simulink model "NL1model"  (R2024a)
settings: Solver=FixedStepAuto  StartTime=0.0  StopTime=100  FixedStep=0.001  RelTol=1e-3  AbsTol=1e-3
libraries: fl_lib x17, nesl_utility x11, simulink x3, sdl_lib x1
settings Model: Creator=sa21280  LastModifiedBy=sa21280
settings SolverCC: AutoScaleAbsTol=off  AlgebraicLoopSolver=TrustRegion  MaxZcPerStep=1
settings DebuggingCC: UnconnectedInputMsg=warning  UnconnectedOutputMsg=warning  UnconnectedLineMsg=warning  SymbolicDimsDataTypeCodeGenerationDiagnostic=none
settings ModelReferenceCC: EnableRefExpFcnMdlSchedulingChecks=on
settings SFSimCC: CustomCodeUndefinedFunction=UseInterfaceOnly
settings RTWCC: GPUComputeCapability=3.5  DLArmComputeVersion=19.05
settings SimscapeCC: SimscapeLogType=all  SimscapeLogSimulationStatistics=on  SimscapeLogDataHistory=10000

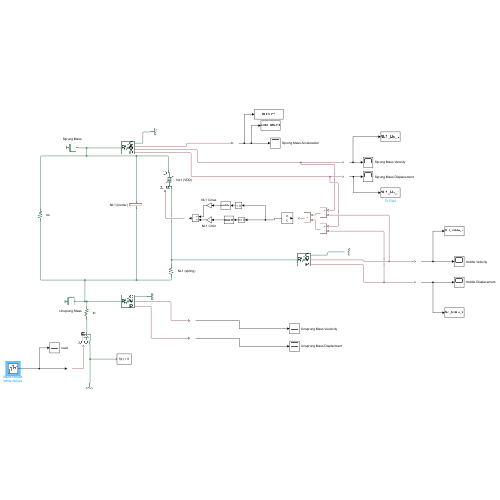
[thumbnail: Simulink's stored preview of the top-level diagram]
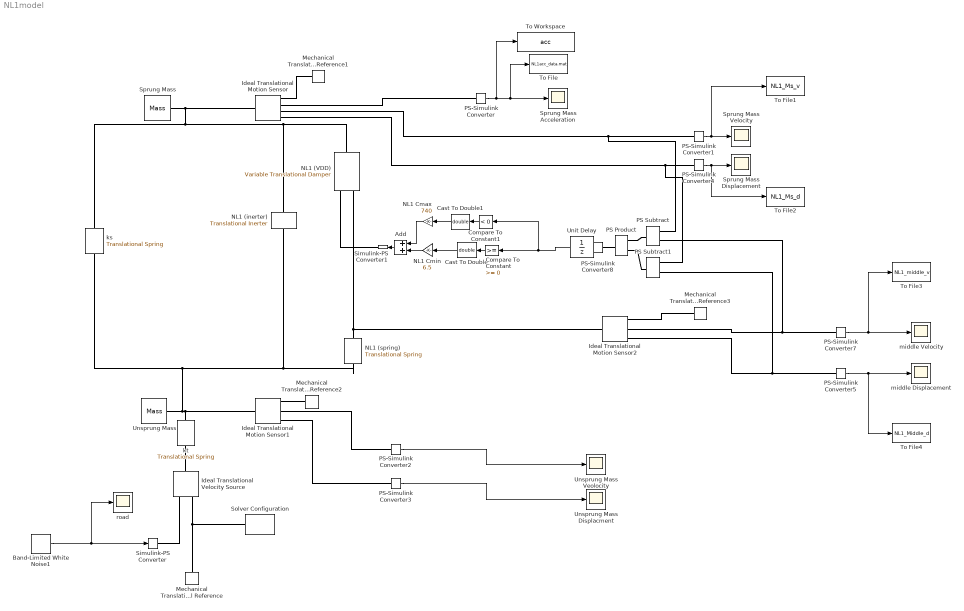
== system NL1model ==
  Add : Sum
  Band-Limited White Noise1 : simulink/Sources/Band-Limited White Noise  Cov=(2*pi*(25*5e-7).^0.5).^2  Ts=0.001  seed=[23341]
  Cast To Double : DataTypeConversion  OutDataTypeStr=double  SaturateOnIntegerOverflow=off  RndMeth=Floor
  Cast To Double1 : DataTypeConversion  OutDataTypeStr=double  SaturateOnIntegerOverflow=off  RndMeth=Floor
  Compare To Constant : simulink/Logic and Bit Operations/Compare To Constant  relop=>=  const=0  OutDataTypeStr=boolean
  Compare To Constant1 : simulink/Logic and Bit Operations/Compare To Constant  relop=<  const=0  OutDataTypeStr=boolean
  Ideal Translational Motion Sensor : fl_lib/Mechanical/Mechanical Sensors/Ideal Translational Motion Sensor  reference=foundation.enum.MeasurementReference.difference  acceleration_port=true  velocity_port=true  position_port=true  offset=0 m
      settings: InternalSimscapePortConfiguration="{\"Bottom\":[],\"Left\":[{\"id\":\"R\",\"label\":\"R\",\"type\":\"foundation.mechanical.translational.translational\"}],\"Right\":[{\"id\":\"C\",\"label\":\"C\",\"type\":\"foundation.mechanical.translational.translational\"},{\"id\":\"A\",\"label\":\"A\",\"type\":\"output\"},{\"id\":\"V\",\"label\":\"V\",\"type\":\"output\"},{\"id\":\"P\",\"label\":\"P\",\"type\":\"output\"}],\"Top\":[]}"
  Ideal Translational Motion Sensor1 : fl_lib/Mechanical/Mechanical Sensors/Ideal Translational Motion Sensor  reference=foundation.enum.MeasurementReference.difference  acceleration_port=false  velocity_port=true  position_port=true  offset=0 m
  Ideal Translational Motion Sensor2 : fl_lib/Mechanical/Mechanical Sensors/Ideal Translational Motion Sensor  reference=foundation.enum.MeasurementReference.difference  acceleration_port=false  velocity_port=true  position_port=true  offset=0 m
  Ideal Translational Velocity Source : fl_lib/Mechanical/Mechanical Sources/Ideal Translational Velocity Source
  Mechanical Translational Reference{,1..3} (4 alike) : fl_lib/Mechanical/Translational Elements/Mechanical Translational Reference
  NL1 (VDD) : sdl_lib/Couplings & Drives/Springs & Dampers/Variable Translational Damper  Bmin=0 N*s/m
      settings: InternalSimscapePortConfiguration="{\"Bottom\":[],\"Left\":[{\"id\":\"B\",\"label\":\"B\",\"type\":\"input\"},{\"id\":\"R\",\"label\":\"R\",\"type\":\"foundation.mechanical.translational.translational\"}],\"Right\":[{\"id\":\"C\",\"label\":\"C\",\"type\":\"foundation.mechanical.translational.translational\"}],\"Top\":[]}"
  NL1 (inerter) : fl_lib/Mechanical/Translational Elements/Translational Inerter  B=6.0625 kg  v_specify=off  v_priority=High  v=0 m/s  v_nominal_specify=off  v_nominal_value=1  v_nominal_unit=m/s  f_specify=off  f_priority=None  f=0 N  f_nominal_specify=off  f_nominal_value=1  f_nominal_unit=N
      settings: InternalSimscapePortConfiguration="{\"Bottom\":[],\"Left\":[{\"id\":\"R\",\"label\":\"R\",\"type\":\"foundation.mechanical.translational.translational\"}],\"Right\":[{\"id\":\"C\",\"label\":\"C\",\"type\":\"foundation.mechanical.translational.translational\"}],\"Top\":[]}"
  NL1 (spring) : fl_lib/Mechanical/Translational Elements/Translational Spring  spr_rate=20000 N/m  v_specify=off  v_priority=None  v=0 m/s  v_nominal_specify=off  v_nominal_value=1  v_nominal_unit=m/s  f_specify=off  f_priority=None  f=0 N  f_nominal_specify=off  f_nominal_value=1  f_nominal_unit=N  x_specify=off  x_priority=High  x=0 m  x_nominal_specify=off  x_nominal_value=1  x_nominal_unit=m
  NL1 Cmax : Gain  Gain=740
  NL1 Cmin : Gain  Gain=6.5
  PS Product : fl_lib/Physical Signals/Functions/PS Product
  PS Subtract : fl_lib/Physical Signals/Functions/PS Subtract
  PS Subtract1 : fl_lib/Physical Signals/Functions/PS Subtract
  PS-Simulink Converter{,1..5,7..8} (8 alike) : nesl_utility/PS-Simulink Converter  PhysicalDomain=network_engine_domain  SubClassName=ps_output  LeftPortType=input  RightPortType=output  PseudoPeriodic=off  Frequencies=[]  VectorFormat=inherit  Unit=inherit  AffineConversion=off
  Simulink-PS Converter : nesl_utility/Simulink-PS Converter  PhysicalDomain=network_engine_domain  SubClassName=ps_input  LeftPortType=input  RightPortType=output  PseudoPeriodic=off  Frequencies=[]  NoiseDistribution=none  NoiseParameters=[]  Unit=1  AffineConversion=off  FilteringAndDerivatives=provide  SimscapeFilterOrder=1  InputFilterTimeConstant=0.001  UdotUserProvided=0
  Simulink-PS Converter1 : nesl_utility/Simulink-PS Converter  PhysicalDomain=network_engine_domain  SubClassName=ps_input  LeftPortType=input  RightPortType=output  PseudoPeriodic=off  Frequencies=[]  NoiseDistribution=none  NoiseParameters=[]  Unit=1  AffineConversion=off  FilteringAndDerivatives=provide  SimscapeFilterOrder=1  InputFilterTimeConstant=0.001  UdotUserProvided=0
  Solver Configuration : nesl_utility/Solver Configuration  PhysicalDomain=network_engine_domain  SubClassName=solver  LeftPortType=input  RightPortType=generic  Tones=[]  Harmonics=[]  SimulateNoise=off  Profile=off  UseLocalSampling=off  EnableSwitchedLinearOptims=on  FrequencyDomain=off  UseCCode=off  RelTol=0.001  AbsTol=0.001  MinStep=1e-09  ToWorkspace=off  RevertToSquareIcSolve=off  NumHomotopyIterations=100  PhasorMode=off  PhasorModeNumHarmonics=1  ConsistencySolver=NEWTON_XTOL_AFTER_FTOL  IndexReductionMethod=DerivativeReplacement  DoDC=off  ResidualTolerance=1e-09  ConsistencyTolSource=GLOBAL  ConsistencyAbsTol=0.001  ConsistencyRelTol=0.001  ConsistencyTolFactor=0.001  UseLocalSolver=off  LocalSolverChoice=NE_BACKWARD_EULER_ADVANCER  ResolveIndetEquations=on  FunctionEvalNumThread=1  LocalSolverSampleTime=0.001  DoFixedCost=off  MaxNonlinIter=3  MaxModeIter=2  ComputeImpulses=off  ImpulseIterations=2  LinearAlgebra=auto  LinearAlgebraNumThread=0  EquationFormulation=NE_TIME_EF  DelaysMemoryBudget=1024  AutomaticFiltering=on  FilteringTimeConstant=0.001  PartitionStorageMethod=AS_NEEDED  PartitionMemoryBudget=1024  PartitionMethod=ROBUST  MultibodyUseLocalSolver=off  MultibodyLocalSolverChoice=ODE1  MultibodyLocalSolverSampleTime=0.001
  Sprung Mass : fl_lib/Mechanical/Translational Elements/Mass  mass=240 kg  num_ports=foundation.enum.numPorts2.one  v_specify=off  v_priority=High  v=0 m/s  v_nominal_specify=off  v_nominal_value=1  v_nominal_unit=m/s  f_specify=off  f_priority=None  f=0 N  f_nominal_specify=off  f_nominal_value=1  f_nominal_unit=N
  Sprung Mass Acceleration : Scope
  Sprung Mass Displacement : Scope
  Sprung Mass Velocity : Scope
  To File : ToFile  Filename=NL1acc_data.mat  MatrixName=Ms_acc  SaveFormat=Timeseries
  To File1 : ToFile  Filename=NL1_Ms_v  MatrixName=Ms_v  SaveFormat=Timeseries
  To File2 : ToFile  Filename=NL1_Ms_d  MatrixName=Ms_d  SaveFormat=Timeseries
  To File3 : ToFile  Filename=NL1_middle_v  MatrixName=middle_v  SaveFormat=Timeseries
  To File4 : ToFile  Filename=NL1_Middle_d  MatrixName=middle_d  SaveFormat=Timeseries
  To Workspace : ToWorkspace  VariableName=acc  SaveFormat=Timeseries  SampleTime=-1
  Unit Delay : UnitDelay  SampleTime=-1  HasFrameUpgradeWarning=on
  Unsprung Mass : fl_lib/Mechanical/Translational Elements/Mass  mass=36 kg  num_ports=foundation.enum.numPorts2.one  v_specify=off  v_priority=High  v=0 m/s  v_nominal_specify=off  v_nominal_value=1  v_nominal_unit=m/s  f_specify=off  f_priority=None  f=0 N  f_nominal_specify=off  f_nominal_value=1  f_nominal_unit=N
  Unsprung Mass Displacment : Scope
  Unsprung Mass Veolocity : Scope
  ks : fl_lib/Mechanical/Translational Elements/Translational Spring  spr_rate=16000 N/m  v_specify=off  v_priority=None  v=0 m/s  v_nominal_specify=off  v_nominal_value=1  v_nominal_unit=m/s  f_specify=off  f_priority=None  f=0 N  f_nominal_specify=off  f_nominal_value=1  f_nominal_unit=N  x_specify=off  x_priority=High  x=0 m  x_nominal_specify=off  x_nominal_value=1  x_nominal_unit=m
  kt : fl_lib/Mechanical/Translational Elements/Translational Spring  spr_rate=160000 N/m  v_specify=off  v_priority=None  v=0 m/s  v_nominal_specify=off  v_nominal_value=1  v_nominal_unit=m/s  f_specify=off  f_priority=None  f=0 N  f_nominal_specify=off  f_nominal_value=1  f_nominal_unit=N  x_specify=off  x_priority=High  x=0 m  x_nominal_specify=off  x_nominal_value=1  x_nominal_unit=m
  "middle Displacement " : Scope
  middle Velocity : Scope
  road : Scope
  wires:
  PS-Simulink Converter/1 -> To Workspace/1, To File/1, Sprung Mass Acceleration/1
  PS-Simulink Converter3/1 -> Unsprung Mass Displacment/1
  PS-Simulink Converter2/1 -> Unsprung Mass Veolocity/1
  Band-Limited White Noise1/1 -> road/1, Simulink-PS Converter/1
  PS-Simulink Converter7/1 -> To File3/1, middle Velocity/1
  PS-Simulink Converter5/1 -> To File4/1, "middle Displacement "/1
  PS-Simulink Converter8/1 -> Unit Delay/1
  Unit Delay/1 -> Compare To Constant/1, Compare To Constant1/1
  NL1 Cmin/1 -> Add/2
  Add/1 -> Simulink-PS Converter1/1
  Cast To Double1/1 -> NL1 Cmax/1
  Compare To Constant1/1 -> Cast To Double1/1
  Compare To Constant/1 -> Cast To Double/1
  Cast To Double/1 -> NL1 Cmin/1
  NL1 Cmax/1 -> Add/1
  PS-Simulink Converter1/1 -> To File1/1, Sprung Mass Velocity/1
  PS-Simulink Converter4/1 -> To File2/1, Sprung Mass Displacement/1
  connections:
  Sprung Mass/LConn1 -- NL1 (inerter)/RConn1 -- NL1 (VDD)/RConn1 -- ks/RConn1 -- Ideal Translational Motion Sensor/LConn1
  Ideal Translational Motion Sensor1/LConn1 -- Unsprung Mass/LConn1 -- NL1 (spring)/LConn1 -- NL1 (inerter)/LConn1 -- ks/LConn1 -- kt/RConn1
  Ideal Translational Velocity Source/LConn1 -- kt/LConn1
  Simulink-PS Converter/RConn1 -- Ideal Translational Velocity Source/RConn1
  Mechanical Translational Reference/LConn1 -- Solver Configuration/RConn1 -- Ideal Translational Velocity Source/RConn2
  PS-Simulink Converter1/LConn1 -- PS Subtract/LConn2 -- Ideal Translational Motion Sensor/RConn3
  Ideal Translational Motion Sensor/RConn2 -- PS-Simulink Converter/LConn1
  Mechanical Translational Reference1/LConn1 -- Ideal Translational Motion Sensor/RConn1
  PS-Simulink Converter3/LConn1 -- Ideal Translational Motion Sensor1/RConn3
  Mechanical Translational Reference2/LConn1 -- Ideal Translational Motion Sensor1/RConn1
  Ideal Translational Motion Sensor1/RConn2 -- PS-Simulink Converter2/LConn1
  PS-Simulink Converter4/LConn1 -- PS Subtract1/LConn2 -- Ideal Translational Motion Sensor/RConn4
  NL1 (spring)/RConn1 -- NL1 (VDD)/LConn2 -- Ideal Translational Motion Sensor2/LConn1
  Mechanical Translational Reference3/LConn1 -- Ideal Translational Motion Sensor2/RConn1
  PS Product/LConn2 -- PS Subtract/RConn1
  PS-Simulink Converter8/LConn1 -- PS Product/RConn1
  PS Product/LConn1 -- PS Subtract1/RConn1
  Simulink-PS Converter1/RConn1 -- NL1 (VDD)/LConn1
  Ideal Translational Motion Sensor2/RConn3 -- PS Subtract1/LConn1 -- PS-Simulink Converter5/LConn1
  Ideal Translational Motion Sensor2/RConn2 -- PS Subtract/LConn1 -- PS-Simulink Converter7/LConn1
